simulink model "simscape_model_Shunt"  (R2023b)
settings: Solver=VariableStepAuto  StartTime=0.0  StopTime=10  RelTol=1e-3
values from neighbouring files (symbols this model uses):
  Bm = 0.000001074    (= 1.074e-06)    [setup_params_shunt.m]
  LAF = 0.004    [setup_params_shunt.m]
  ra = 0.013    [setup_params_shunt.m]
  rf = 1.43    [setup_params_shunt.m]
  Tl = 2.493    [setup_params_shunt.m]
  Va = 24    [setup_params_shunt.m]
libraries: fl_lib x15, nesl_utility x10
settings Model: Creator=Noor  LastModifiedBy=USER
settings SolverCC: AlgebraicLoopSolver=TrustRegion
settings DataIOCC: ReturnWorkspaceOutputs=off
settings DebuggingCC: UnconnectedInputMsg=warning  UnconnectedOutputMsg=warning  UnconnectedLineMsg=warning  ArithmeticOperatorsInVariantConditions=warning
settings ModelReferenceCC: EnableRefExpFcnMdlSchedulingChecks=on
settings SFSimCC: SimUseLocalCustomCode=off  CustomCodeUndefinedFunction=UseInterfaceOnly
settings RTWCC: RTWUseLocalCustomCode=off

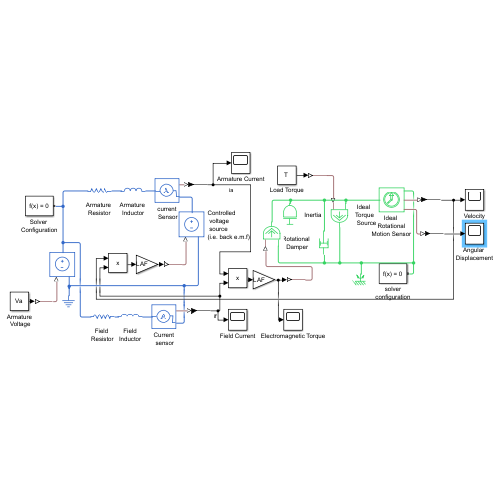
[thumbnail: Simulink's stored preview of the top-level diagram]
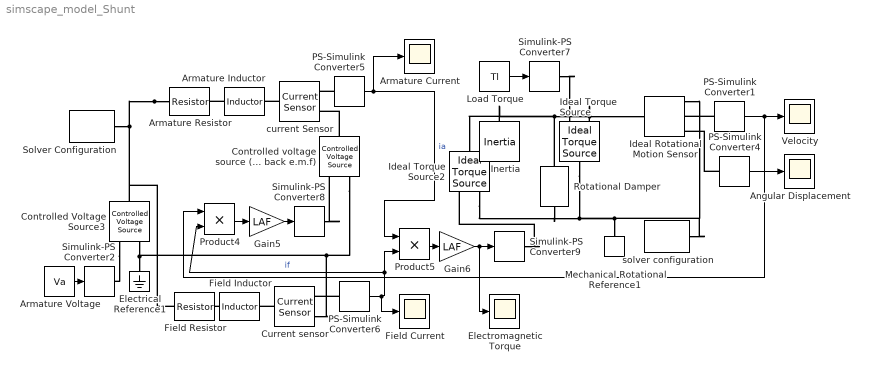
== system simscape_model_Shunt ==
  " Ideal Torque Source" : fl_lib/Mechanical/Mechanical Sources/Ideal Torque Source
  Angular Displacement : Scope
  Armature Voltage : Constant  Value=Va
  Armature Inductor : fl_lib/Electrical/Electrical Elements/Inductor  l=LAA H  r=0 Ohm  g=0 1/Ohm  i_specify=off  i_priority=None  i=0 A  i_nominal_specify=off  i_nominal_unit=A  i_nominal_value=1  v_specify=off  v_priority=None  v=0 V  v_nominal_specify=off  v_nominal_unit=V  v_nominal_value=1  i_L_specify=off  i_L_priority=High  i_L=0 A  i_L_nominal_specify=off  i_L_nominal_unit=A  i_L_nominal_value=1
  Armature Resistor : fl_lib/Electrical/Electrical Elements/Resistor  R=ra Ohm  i_specify=off  i_priority=None  i=0 A  i_nominal_specify=off  i_nominal_unit=A  i_nominal_value=1  v_specify=off  v_priority=None  v=0 V  v_nominal_specify=off  v_nominal_unit=V  v_nominal_value=1
  Armature Current : Scope
  Controlled voltage source (i.e. back e.m.f) : fl_lib/Electrical/Electrical Sources/Controlled Voltage Source
  Controlled Voltage Source3 : fl_lib/Electrical/Electrical Sources/Controlled Voltage Source
  Current sensor : fl_lib/Electrical/Electrical Sensors/Current Sensor
  Electrical Reference1 : fl_lib/Electrical/Electrical Elements/Electrical Reference
  Electromagnetic Torque : Scope
  Field Inductor : fl_lib/Electrical/Electrical Elements/Inductor  l=LFF H  r=0 Ohm  g=0 1/Ohm  i_specify=off  i_priority=None  i=0 A  i_nominal_specify=off  i_nominal_unit=A  i_nominal_value=1  v_specify=off  v_priority=None  v=0 V  v_nominal_specify=off  v_nominal_unit=V  v_nominal_value=1  i_L_specify=off  i_L_priority=High  i_L=0 A  i_L_nominal_specify=off  i_L_nominal_unit=A  i_L_nominal_value=1
  Field Resistor : fl_lib/Electrical/Electrical Elements/Resistor  R=rf Ohm  i_specify=off  i_priority=None  i=0 A  i_nominal_specify=off  i_nominal_unit=A  i_nominal_value=1  v_specify=off  v_priority=None  v=0 V  v_nominal_specify=off  v_nominal_unit=V  v_nominal_value=1
  Field Current : Scope
  Gain5 : Gain  Gain=LAF
  Gain6 : Gain  Gain=LAF
  Ideal Rotational Motion Sensor : fl_lib/Mechanical/Mechanical Sensors/Ideal Rotational Motion Sensor  reference=foundation.enum.MeasurementReference.difference  acceleration_port=false  velocity_port=true  position_port=true  wrap_angle=false  offset=0 rev
  Ideal Torque Source2 : fl_lib/Mechanical/Mechanical Sources/Ideal Torque Source
  "Inertia " : fl_lib/Mechanical/Rotational Elements/Inertia  inertia=J kg*m^2  num_ports=foundation.enum.numPorts2.one  w_specify=off  w_priority=High  w=0 rad/s  w_nominal_specify=off  w_nominal_unit=rad/s  w_nominal_value=1  t_specify=off  t_priority=None  t=0 N*m  t_nominal_specify=off  t_nominal_unit=N*m  t_nominal_value=1
  Load Torque : Constant  Value=Tl
  Mechanical Rotational Reference1 : fl_lib/Mechanical/Rotational Elements/Mechanical Rotational Reference
  PS-Simulink Converter{1,4..6} (4 alike) : nesl_utility/PS-Simulink Converter  PhysicalDomain=network_engine_domain  SubClassName=ps_output  LeftPortType=input  RightPortType=output  PseudoPeriodic=off  Frequencies=[]  VectorFormat=1-D array  Unit=1  AffineConversion=off
  Product4 : Product
  Product5 : Product
  "Rotational Damper  " : fl_lib/Mechanical/Rotational Elements/Rotational Damper  D=Bm N*m/(rad/s)  w_specify=off  w_priority=None  w=0 rad/s  w_nominal_specify=off  w_nominal_unit=rad/s  w_nominal_value=1  t_specify=off  t_priority=None  t=0 N*m  t_nominal_specify=off  t_nominal_unit=N*m  t_nominal_value=1
  Simulink-PS Converter{2,7..9} (4 alike) : nesl_utility/Simulink-PS Converter  PhysicalDomain=network_engine_domain  SubClassName=ps_input  LeftPortType=input  RightPortType=output  PseudoPeriodic=off  Frequencies=[]  NoiseDistribution=none  NoiseParameters=[]  Unit=1  AffineConversion=off  FilteringAndDerivatives=provide  SimscapeFilterOrder=1  InputFilterTimeConstant=0.001  UdotUserProvided=0
  Solver Configuration : nesl_utility/Solver Configuration  PhysicalDomain=network_engine_domain  SubClassName=solver  LeftPortType=input  RightPortType=generic  Tones=[]  Harmonics=[]  SimulateNoise=off  Profile=off  UseLocalSampling=off  EnableSwitchedLinearOptims=on  FrequencyDomain=off  UseCCode=off  RelTol=0.001  AbsTol=1e-06  MinStep=1e-09  ToWorkspace=off  RevertToSquareIcSolve=off  NumHomotopyIterations=100  PhasorMode=off  PhasorModeNumHarmonics=1  ConsistencySolver=NEWTON_FTOL  IndexReductionMethod=DerivativeReplacement  DoDC=off  ResidualTolerance=1e-09  ConsistencyTolSource=GLOBAL  ConsistencyAbsTol=0.001  ConsistencyRelTol=0.001  ConsistencyTolFactor=0.001  UseLocalSolver=off  LocalSolverChoice=NE_BACKWARD_EULER_ADVANCER  ResolveIndetEquations=on  FunctionEvalNumThread=1  LocalSolverSampleTime=0.001  DoFixedCost=off  MaxNonlinIter=3  MaxModeIter=2  ComputeImpulses=off  ImpulseIterations=2  LinearAlgebra=Sparse  LinearAlgebraNumThread=0  EquationFormulation=NE_TIME_EF  DelaysMemoryBudget=1024  AutomaticFiltering=on  FilteringTimeConstant=0.001  PartitionStorageMethod=AS_NEEDED  PartitionMemoryBudget=1024  PartitionMethod=FAST  MultibodyUseLocalSolver=off  MultibodyLocalSolverChoice=ODE1  MultibodyLocalSolverSampleTime=0.001
  Velocity : Scope
  "current Sensor " : fl_lib/Electrical/Electrical Sensors/Current Sensor
  solver configuration : nesl_utility/Solver Configuration  PhysicalDomain=network_engine_domain  SubClassName=solver  LeftPortType=input  RightPortType=generic  Tones=[]  Harmonics=[]  SimulateNoise=off  Profile=off  UseLocalSampling=off  EnableSwitchedLinearOptims=on  FrequencyDomain=off  UseCCode=off  RelTol=0.001  AbsTol=1e-06  MinStep=1e-09  ToWorkspace=off  RevertToSquareIcSolve=off  NumHomotopyIterations=100  PhasorMode=off  PhasorModeNumHarmonics=1  ConsistencySolver=NEWTON_FTOL  IndexReductionMethod=DerivativeReplacement  DoDC=off  ResidualTolerance=1e-09  ConsistencyTolSource=GLOBAL  ConsistencyAbsTol=0.001  ConsistencyRelTol=0.001  ConsistencyTolFactor=0.001  UseLocalSolver=off  LocalSolverChoice=NE_BACKWARD_EULER_ADVANCER  ResolveIndetEquations=on  FunctionEvalNumThread=1  LocalSolverSampleTime=0.001  DoFixedCost=off  MaxNonlinIter=3  MaxModeIter=2  ComputeImpulses=off  ImpulseIterations=2  LinearAlgebra=Sparse  LinearAlgebraNumThread=0  EquationFormulation=NE_TIME_EF  DelaysMemoryBudget=1024  AutomaticFiltering=on  FilteringTimeConstant=0.001  PartitionStorageMethod=AS_NEEDED  PartitionMemoryBudget=1024  PartitionMethod=FAST  MultibodyUseLocalSolver=off  MultibodyLocalSolverChoice=ODE1  MultibodyLocalSolverSampleTime=0.001
  wires:
  PS-Simulink Converter4/1 -> Angular Displacement/1
  Armature Voltage/1 -> Simulink-PS Converter2/1
  Product5/1 -> Gain6/1
  Product4/1 -> Gain5/1
  PS-Simulink Converter1/1 -> Product4/1, Velocity/1
  Load Torque/1 -> Simulink-PS Converter7/1
  PS-Simulink Converter5/1 -> Armature Current/1, Product5/1  "ia"
  Gain6/1 -> Electromagnetic Torque/1, Simulink-PS Converter9/1
  Gain5/1 -> Simulink-PS Converter8/1
  PS-Simulink Converter6/1 -> Product5/2, Product4/2, Field Current/1  "if"
  connections:
  " Ideal Torque Source"/RConn2 -- Ideal Torque Source2/LConn1 -- "Inertia "/LConn1 -- "Rotational Damper  "/LConn1 -- Ideal Rotational Motion Sensor/LConn1
  " Ideal Torque Source"/LConn1 -- "Rotational Damper  "/RConn1 -- Ideal Torque Source2/RConn2 -- Ideal Rotational Motion Sensor/RConn1 -- solver configuration/RConn1 -- Mechanical Rotational Reference1/LConn1
  Controlled voltage source (i.e. back e.m.f)/RConn2 -- Current sensor/RConn2 -- Controlled Voltage Source3/RConn2 -- Electrical Reference1/LConn1
  Armature Resistor/LConn1 -- Field Resistor/LConn1 -- Controlled Voltage Source3/LConn1 -- Solver Configuration/RConn1
  PS-Simulink Converter4/LConn1 -- Ideal Rotational Motion Sensor/RConn3
  Controlled voltage source (i.e. back e.m.f)/LConn1 -- "current Sensor "/RConn2
  PS-Simulink Converter1/LConn1 -- Ideal Rotational Motion Sensor/RConn2
  Simulink-PS Converter9/RConn1 -- Ideal Torque Source2/RConn1
  PS-Simulink Converter5/LConn1 -- "current Sensor "/RConn1
  Field Inductor/LConn1 -- Field Resistor/RConn1
  Simulink-PS Converter8/RConn1 -- Controlled voltage source (i.e. back e.m.f)/RConn1
  Simulink-PS Converter7/RConn1 -- " Ideal Torque Source"/RConn1
  Armature Inductor/LConn1 -- Armature Resistor/RConn1
  Controlled Voltage Source3/RConn1 -- Simulink-PS Converter2/RConn1
  "current Sensor "/LConn1 -- Armature Inductor/RConn1
  PS-Simulink Converter6/LConn1 -- Current sensor/RConn1
  Current sensor/LConn1 -- Field Inductor/RConn1
